simulink model "full_system_phase_control_dq0"  (R2015b)
settings: Solver=VariableStepAuto  StartTime=0.0  StopTime=10  FixedStep=T  RelTol=1e-2
values from neighbouring files (symbols this model uses):
  c_drag_pro = c_drag*G1.^3*r.^3/G2.^3    [Parameters.m]
  G1 = 12    [Parameters.m]
  G2 = 50    [Parameters.m]
  J_M = 52e-4    (= 0.0052)    [Parameters.m]
  J_pro = (m*r^2+J_G2)*(G1/G2)^2 + J_G1    (= 0.281547798877)    [Parameters.m]
  Ki = (3*alpha^2-((Kp*Kv)/(2*J_pro)-(Kv*R)/(J_pro*L)-(3*Kt^2)/(2*J_pro*L)))*L    (= 1.75664037993)    [Parameters.m]
  Kp = (3*alpha-Kv/J_pro-(R/(2*L)))*L    (= 0.0111498579282)    [Parameters.m]
  Kt = .07329    (= 0.07329)    [Parameters.m]
  L = 4e-5    (= 4e-05)    [Parameters.m]
  N = 4    [Parameters.m]
  r = 11*.0254/2    (= 0.1397)    [Parameters.m]
undefined symbols (not defined in the file or in its folder): sigbuilder_block
libraries: fl_lib x19, nesl_utility x10, pe_lib x2, powerlib_meascontrol x2
settings Model: Creator=Martin Andersen  LastModifiedBy=Martin Andersen
settings SolverCC: AlgebraicLoopSolver=LineSearch

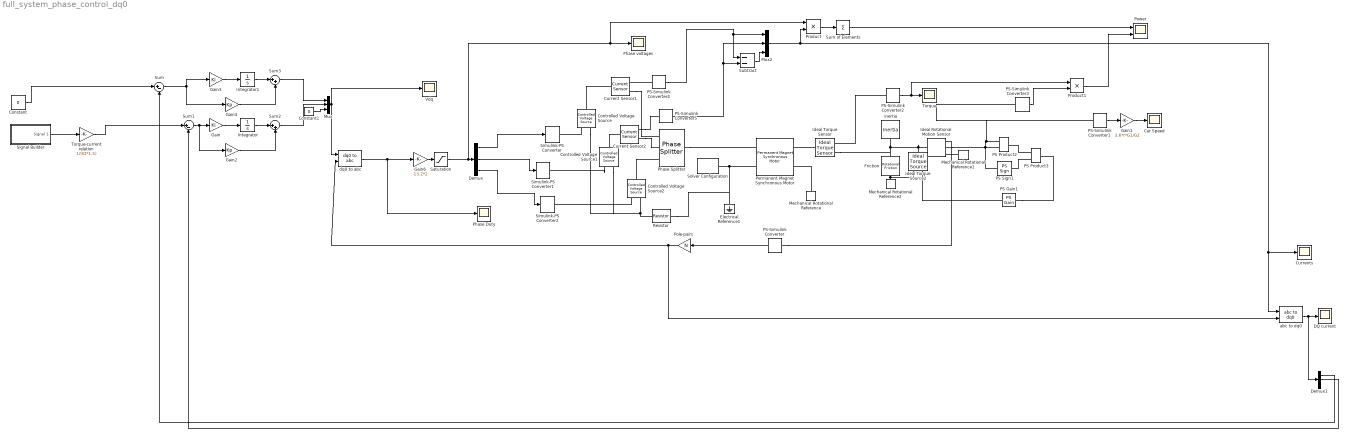
== system full_system_phase_control_dq0 ==
  Car Speed : Scope
  Constant : Constant  Value=0
  Constant1 : Constant  Value=0
  Controlled Voltage Source : fl_lib/Electrical/Electrical Sources/Controlled Voltage Source
  Controlled Voltage Source1 : fl_lib/Electrical/Electrical Sources/Controlled Voltage Source
  Controlled Voltage Source2 : fl_lib/Electrical/Electrical Sources/Controlled Voltage Source
  Current Sensor1 : fl_lib/Electrical/Electrical Sensors/Current Sensor
  Current Sensor2 : fl_lib/Electrical/Electrical Sensors/Current Sensor
  Currents : Scope
  DQ current : Scope
  Demux : Demux  Outputs=3
  Demux1 : Demux  Outputs=3
  Electrical Reference1 : fl_lib/Electrical/Electrical Elements/Electrical Reference
  Friction : fl_lib/Mechanical/Rotational Elements/Rotational Friction  brkwy_trq=.5 N*m  Col_trq=.05 N*m  visc_coef=0.00001 N*m/(rad/s)  trans_coef=10 s/rad  vel_thr=1e-4 rad/s  w_specify=off  w_priority=None  w=0 rad/s  t_specify=off  t_priority=None  t=0 N*m
  Gain : Gain  Gain=Ki
  Gain1 : Gain  Gain=3.6*r*G1/G2
  Gain2 : Gain  Gain=Kp
  Gain3 : Gain  Gain=Ki
  Gain4 : Gain  Gain=Kp
  Gain6 : Gain  Gain=13.2*2
  Ideal Rotational Motion Sensor : fl_lib/Mechanical/Mechanical Sensors/Ideal Rotational Motion Sensor  offset=0 rad
  Ideal Torque Sensor : fl_lib/Mechanical/Mechanical Sensors/Ideal Torque Sensor
  Ideal Torque Source2 : fl_lib/Mechanical/Mechanical Sources/Ideal Torque Source
  Integrator : Integrator  LimitOutput=on  UpperSaturationLimit=1  LowerSaturationLimit=-1
  Integrator1 : Integrator  LimitOutput=on  UpperSaturationLimit=1  LowerSaturationLimit=-1
  Mechanical Rotational Reference : fl_lib/Mechanical/Rotational Elements/Mechanical Rotational Reference
  Mechanical Rotational Reference1 : fl_lib/Mechanical/Rotational Elements/Mechanical Rotational Reference
  Mechanical Rotational Reference2 : fl_lib/Mechanical/Rotational Elements/Mechanical Rotational Reference
  Mux : Mux  Inputs=3
  Mux2 : Mux  Inputs=3
  PS Gain1 : fl_lib/Physical Signals/Functions/PS Gain  gain=c_drag_pro
  PS Product2 : fl_lib/Physical Signals/Functions/PS Product
  PS Product3 : fl_lib/Physical Signals/Functions/PS Product
  PS Sign1 : fl_lib/Physical Signals/Nonlinear Operators/PS Sign
  PS-Simulink Converter{,1..5} (6 alike) : nesl_utility/PS-Simulink Converter  PhysicalDomain=network_engine_domain  SubClassName=ps_output  LeftPortType=input  RightPortType=output  PseudoPeriodic=off  Frequencies=[]  Unit=1  AffineConversion=off
  Permanent Magnet Synchronous Motor : pe_lib/Machines/Permanent Magnet Rotor/Permanent Magnet Synchronous Motor  nPolePairs=N  pm_flux_linkage=Kt/N Wb  stator_param=1  Ld=L H  Lq=L H  L0=L H  Ls=L H  Lm=0 H  Ms=L/10 H  Rs=R Ohm  initial_currents=[0, 0, 0] A  axes_param=2  angular_position0=0 rad  rotor_offset=- pi / 2 rad  shift_3ph=[nan, nan, nan] rad  sqrt2OverSqrt3=nan  oneOverSqrt2=nan  twoPiOver3=nan  Lmin=1e-9 H
  Phase Duty : Scope
  Phase Splitter : pe_lib/Connections/Phase Splitter
  Phase voltages : Scope
  Pole-pairs : Gain  Gain=N
  Power : Scope  NumInputPorts=2
  Product : Product
  Product1 : Product
  Resistor : fl_lib/Electrical/Electrical Elements/Resistor  R=1e9 Ohm  i_specify=off  i_priority=None  i=0 A  v_specify=off  v_priority=None  v=0 V
  Saturation : Saturate  UpperLimit=13.2*2  LowerLimit=-13.2*2
  Signal Builder : Subsystem  Tag=STV Subsys  LoadFcn=sigbuilder_block('load');  StartFcn=sigbuilder_block('start');  StopFcn=sigbuilder_block('stop');  ClipboardFcn=sigbuilder_block('clipboard');  mask(Sigbuilder block){}
      mask help: Simulink:masks:SigbuilderBlock_MD
      mask init:
      | if ~strcmp(get_param(bdroot(gcbh),'SimulationStatus'),'stopped') tuvar = sigbuilder_block('maskInit'); end
      settings: CopyFcn=sigbuilder_block('copy');  DeleteFcn=sigbuilder_block('delete');  ModelCloseFcn=sigbuilder_block('modelClose');  PreSaveFcn=sigbuilder_block('preSave');  PauseFcn=sigbuilder_block('pause');  ContinueFcn=sigbuilder_block('continue');  NameChangeFcn=sigbuilder_block('namechange');  OpenFcn=sigbuilder_block('open',[5.4 30 1141.2 522.6 ]);  CloseFcn=sigbuilder_block('close');
      mask Display: plot(0, 0, 100, 100,[2, 2, 32, 32, 2], [68, 8, 8, 68, 68],[32, 2], [38, 38], [32, 19, 2],[53, 60, 44], [32, 17, 17, 2],[16, 16, 31, 31]);txt = getActiveGroup(gcbh);text(2, 100, txt,'verticalAlignment', 'top');
  Simulink-PS Converter : nesl_utility/Simulink-PS Converter  PhysicalDomain=network_engine_domain  SubClassName=ps_input  LeftPortType=input  RightPortType=output  PseudoPeriodic=off  Frequencies=[]  NoiseDistribution=none  NoiseParameters=[]  Unit=1  AffineConversion=off  InputFiltering=off  SimscapeFilterOrder=1  InputFilterTimeConstant=0.001  UdotUserProvided=1
  Simulink-PS Converter1 : nesl_utility/Simulink-PS Converter  PhysicalDomain=network_engine_domain  SubClassName=ps_input  LeftPortType=input  RightPortType=output  PseudoPeriodic=off  Frequencies=[]  NoiseDistribution=none  NoiseParameters=[]  Unit=1  AffineConversion=off  InputFiltering=off  SimscapeFilterOrder=1  InputFilterTimeConstant=0.001  UdotUserProvided=1
  Simulink-PS Converter2 : nesl_utility/Simulink-PS Converter  PhysicalDomain=network_engine_domain  SubClassName=ps_input  LeftPortType=input  RightPortType=output  PseudoPeriodic=off  Frequencies=[]  NoiseDistribution=none  NoiseParameters=[]  Unit=1  AffineConversion=off  InputFiltering=off  SimscapeFilterOrder=1  InputFilterTimeConstant=0.001  UdotUserProvided=1
  Solver Configuration : nesl_utility/Solver Configuration  PhysicalDomain=network_engine_domain  SubClassName=solver  LeftPortType=input  RightPortType=generic  Accelerate=off  Tones=[]  Harmonics=[]  SimulateNoise=off  Profile=off  UseLocalSampling=off  EnableSwitchedLinearOptims=on  FrequencyDomain=off  UseCCode=off  RelTol=0.001  AbsTol=1e-06  MinStep=1e-09  ToWorkspace=off  RevertToSquareIcSolve=off  NumHomotopyIterations=100  PhasorMode=off  PhasorModeNumHarmonics=1  DoDC=off  ResidualTolerance=1e-9  UseLocalSolver=off  LocalSolverChoice=NE_TRAPEZOIDAL_ADVANCER  LocalSolverSampleTime=0.00001  DoFixedCost=off  MaxNonlinIter=3  MaxModeIter=2  LinearAlgebra=Sparse  DelaysMemoryBudget=102400  AutomaticFiltering=on  FilteringTimeConstant=0.001
  Subtract : Sum  Inputs=--
  Sum : Sum  Inputs=|+-
  Sum of Elements : Sum  Inputs=+
  Sum1 : Sum  Inputs=|+-
  Sum2 : Sum  Inputs=|++
  Sum3 : Sum  Inputs=|++
  Torque : Scope
  Torque-current relation : Gain  Gain=1/(Kt*1.5)
  Vdq : Scope
  abc to dq0 : powerlib_meascontrol/Transformations/abc to dq0  Alignment=Aligned with phase A axis
  dq0 to abc : powerlib_meascontrol/Transformations/dq0 to abc  Alignment=Aligned with phase A axis
  inertia : fl_lib/Mechanical/Rotational Elements/Inertia  inertia=J_M + J_pro kg*m^2  w_specify=off  w_priority=None  w=0 rad/s  t_specify=off  t_priority=None  t=0 N*m
  wires:
  Demux/1 -> Simulink-PS Converter/1
  Demux/2 -> Simulink-PS Converter1/1
  Demux/3 -> Simulink-PS Converter2/1
  PS-Simulink Converter1/1 -> Gain1/1
  Gain1/1 -> Car Speed/1
  PS-Simulink Converter4/1 -> Mux2/1, Subtract/1
  PS-Simulink Converter5/1 -> Mux2/2, Subtract/2
  Saturation/1 -> Product/1, Phase voltages/1, Demux/1
  Mux2/1 -> Product/2, abc to dq0/1, Currents/1
  Subtract/1 -> Mux2/3
  abc to dq0/1 -> Demux1/1, DQ current/1
  PS-Simulink Converter2/1 -> Product1/1, Torque/1
  Product/1 -> Sum of Elements/1
  Sum of Elements/1 -> Power/1
  PS-Simulink Converter3/1 -> Product1/2
  Product1/1 -> Power/2
  Gain6/1 -> Saturation/1
  Pole-pairs/1 -> abc to dq0/2, dq0 to abc/2
  Constant/1 -> Sum/1
  Demux1/1 -> Sum/2
  Demux1/2 -> Sum1/2
  Gain/1 -> Integrator/1
  Sum1/1 -> Gain2/1, Gain/1
  Signal Builder/1(Signal 1) -> Torque-current relation/1
  Integrator/1 -> Sum2/1
  Gain2/1 -> Sum2/2
  Gain3/1 -> Integrator1/1
  Sum/1 -> Gain4/1, Gain3/1
  Integrator1/1 -> Sum3/1
  Gain4/1 -> Sum3/2
  Sum3/1 -> Mux/1
  Sum2/1 -> Mux/2
  Constant1/1 -> Mux/3
  Torque-current relation/1 -> Sum1/1
  Mux/1 -> Vdq/1, dq0 to abc/1
  PS-Simulink Converter/1 -> Pole-pairs/1
  dq0 to abc/1 -> Phase Duty/1, Gain6/1
  connections:
  Permanent Magnet Synchronous Motor/LConn2 -- Resistor/RConn1 -- Electrical Reference1/LConn1 -- Solver Configuration/RConn1
  Mechanical Rotational Reference/LConn1 -- Permanent Magnet Synchronous Motor/RConn2
  PS-Simulink Converter/LConn1 -- Ideal Rotational Motion Sensor/RConn3
  Controlled Voltage Source/RConn1 -- Simulink-PS Converter/RConn1
  Controlled Voltage Source1/RConn1 -- Simulink-PS Converter1/RConn1
  Controlled Voltage Source2/RConn1 -- Simulink-PS Converter2/RConn1
  Controlled Voltage Source2/LConn1 -- Phase Splitter/RConn3
  Controlled Voltage Source1/RConn2 -- Controlled Voltage Source/RConn2 -- Resistor/LConn1 -- Controlled Voltage Source2/RConn2
  Phase Splitter/LConn1 -- Permanent Magnet Synchronous Motor/LConn1
  Current Sensor1/LConn1 -- Controlled Voltage Source/LConn1
  Current Sensor1/RConn2 -- Phase Splitter/RConn1
  Current Sensor2/LConn1 -- Controlled Voltage Source1/LConn1
  Current Sensor2/RConn2 -- Phase Splitter/RConn2
  PS-Simulink Converter4/LConn1 -- Current Sensor1/RConn1
  Current Sensor2/RConn1 -- PS-Simulink Converter5/LConn1
  Ideal Torque Sensor/LConn1 -- Permanent Magnet Synchronous Motor/RConn1
  PS-Simulink Converter2/LConn1 -- Ideal Torque Sensor/RConn2
  Mechanical Rotational Reference2/LConn1 -- Ideal Torque Source2/RConn2 -- Friction/RConn1
  PS Sign1/LConn1 -- PS-Simulink Converter3/LConn1 -- PS-Simulink Converter1/LConn1 -- PS Product2/LConn1 -- Ideal Rotational Motion Sensor/RConn2 -- PS Product2/LConn2
  Ideal Torque Source2/RConn1 -- PS Gain1/RConn1
  PS Product3/LConn2 -- PS Sign1/RConn1
  PS Product3/LConn1 -- PS Product2/RConn1
  PS Gain1/LConn1 -- PS Product3/RConn1
  Mechanical Rotational Reference1/LConn1 -- Ideal Rotational Motion Sensor/RConn1
  Ideal Torque Source2/LConn1 -- inertia/LConn1 -- Ideal Torque Sensor/RConn1 -- Friction/LConn1 -- Ideal Rotational Motion Sensor/LConn1

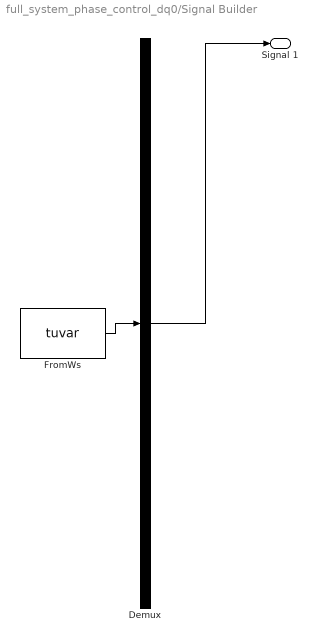
== system full_system_phase_control_dq0/Signal Builder ==
  Demux : Demux  Tag=STV Demux  Outputs=1
  FromWs : FromWorkspace  Tag=STV FromWs  VariableName=tuvar  SampleTime=0
      SigBuilderData=|
      | common.afterFinalStr = 'Extrapolate'
      | common.sampleTime = 0
      | dataSet.timeRange = [0 10]
      | dataSet.name = 'Group 1'
      | sbobj.Groups.Name = 'Group 1'
      | sbobj.Groups.Signals.Name = 'Signal 1'
      | sbobj.Groups.Signals.XData = [0 0.1 0.12 3.49 3.8 10]
      | sbobj.Groups.Signals.YData = [0 0 30.4 32.1 3 1]
  Signal 1 : Outport  Tag=STV Outport
  wires:
  Demux/1 -> Signal 1/1
  FromWs/1 -> Demux/1
